simulink model "simulink2"  (R2017a)
settings: Solver=VariableStepAuto  StartTime=0.0  StopTime=8  RelTol=1e-3
libraries: cstblocks x4
settings Model: Creator=Night_Fury  LastModifiedBy=Havoc

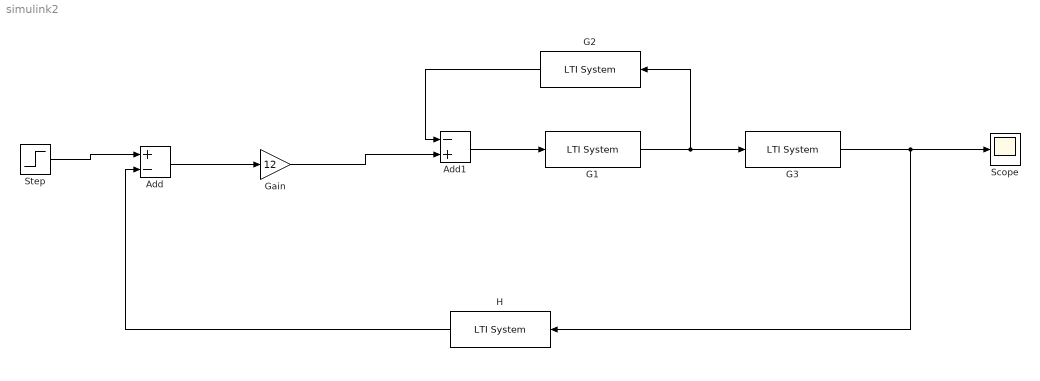
== system simulink2 ==
  Add : Sum  Inputs=+-
  Add1 : Sum  Inputs=-+
  G1 : cstblocks/LTI System  sys=tf(1,[1 1])  IC=[]
  G2 : cstblocks/LTI System  sys=tf(1,[1 1 8])  IC=[]
  G3 : cstblocks/LTI System  sys=tf(20,[1 1])  IC=[]
  Gain : Gain  Gain=12
  H : cstblocks/LTI System  sys=tf(5,[1 0])  IC=[]
  Scope : Scope
  Step : Step  Time=0  SampleTime=0
  wires:
  H/1 -> Add/2
  Step/1 -> Add/1
  G2/1 -> Add1/1
  Add1/1 -> G1/1
  G1/1 -> G2/1, G3/1
  G3/1 -> H/1, Scope/1
  Add/1 -> Gain/1
  Gain/1 -> Add1/2
